simulink model "fdatool8"  (Simulink 5.1)
settings: Solver=FixedStepDiscrete  StartTime=0.0  StopTime=0.5  RelTol=1e-3
libraries: dspsigops x8, fixpt_lib_4 x8
settings Model: Creator=svenhoffmann  LastModifiedBy=svenhoffmann  ExtModeAutoUpdateStatusClock=off  BooleanDataType=on  ProdHWDeviceType=Microprocessor

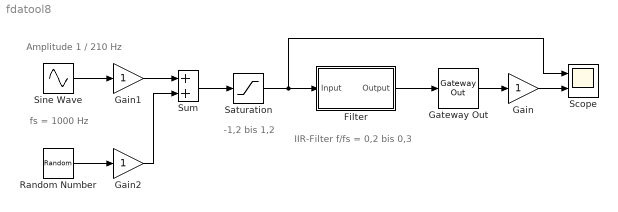
== system fdatool8 ==
  note: IIR-Filter
      | f/fs = 0,2 bis 0,3
  note: Amplitude 1 / 210 Hz
  note: fs = 1000 Hz
  note: -1,2 bis 1,2
  Filter : Subsystem  Tag=FilterWizardSubSystem
  Gain : Gain  SaturateOnIntegerOverflow=on
  Gain1 : Gain  SaturateOnIntegerOverflow=on
  Gain2 : Gain  SaturateOnIntegerOverflow=on
  Gateway Out : fixpt_lib_4/Data Type/Gateway Out  OutRealWorld=Real World Value  OutBuiltInType=double  DoSatur=off
  Random Number : RandomNumber  SampleTime=1/1000
  Saturation : Saturate  UpperLimit=1.2  LowerLimit=-1.2
  Scope : Scope  NumInputPorts=2
      settings: YMin=-5~-5  YMax=5~5
  Sine Wave : Sin  Frequency=2*pi*230  SampleTime=1/1000
  Sum : Sum  SaturateOnIntegerOverflow=on
  wires:
  Sine Wave/1 -> Gain1/1
  Gain/1 -> Scope/2
  Gateway Out/1 -> Gain/1
  Gain1/1 -> Sum/1
  Sum/1 -> Saturation/1
  Random Number/1 -> Gain2/1
  Gain2/1 -> Sum/2
  Saturation/1 -> Scope/1, Filter/1(Input)
  Filter/1(Output) -> Gateway Out/1

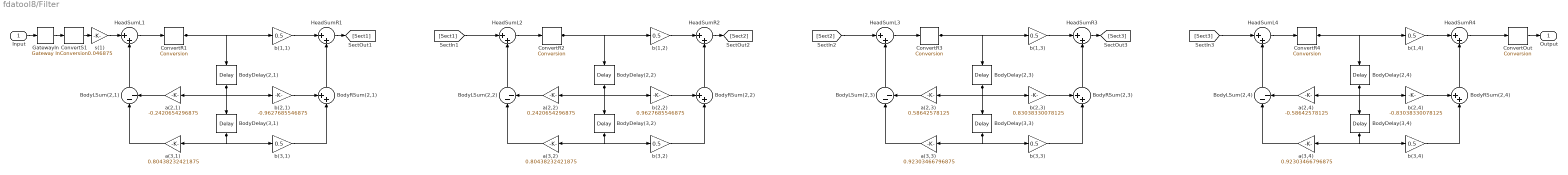
== system fdatool8/Filter ==
  Input : Inport
  BodyDelay(2,1) : dspsigops/Delay  Orientation=down  dly_unit=Samples  delay=1  ic_detail=off  dif_ic_for_ch=off  dif_ic_for_dly=off  ic=0  reset_popup=None
  BodyDelay(2,2) : dspsigops/Delay  Orientation=down  dly_unit=Samples  delay=1  ic_detail=off  dif_ic_for_ch=off  dif_ic_for_dly=off  ic=0  reset_popup=None
  BodyDelay(2,3) : dspsigops/Delay  Orientation=down  dly_unit=Samples  delay=1  ic_detail=off  dif_ic_for_ch=off  dif_ic_for_dly=off  ic=0  reset_popup=None
  BodyDelay(2,4) : dspsigops/Delay  Orientation=down  dly_unit=Samples  delay=1  ic_detail=off  dif_ic_for_ch=off  dif_ic_for_dly=off  ic=0  reset_popup=None
  BodyDelay(3,1) : dspsigops/Delay  Orientation=down  dly_unit=Samples  delay=1  ic_detail=off  dif_ic_for_ch=off  dif_ic_for_dly=off  ic=0  reset_popup=None
  BodyDelay(3,2) : dspsigops/Delay  Orientation=down  dly_unit=Samples  delay=1  ic_detail=off  dif_ic_for_ch=off  dif_ic_for_dly=off  ic=0  reset_popup=None
  BodyDelay(3,3) : dspsigops/Delay  Orientation=down  dly_unit=Samples  delay=1  ic_detail=off  dif_ic_for_ch=off  dif_ic_for_dly=off  ic=0  reset_popup=None
  BodyDelay(3,4) : dspsigops/Delay  Orientation=down  dly_unit=Samples  delay=1  ic_detail=off  dif_ic_for_ch=off  dif_ic_for_dly=off  ic=0  reset_popup=None
  BodyLSum(2,1) : Sum  Orientation=up  Inputs=|--  ShowAdditionalParam=on  OutDataTypeMode=Specify via dialog  OutDataType=sfix(32)  OutScaling=2^-28  SaturateOnIntegerOverflow=on  LockScale=on
  BodyLSum(2,2) : Sum  Orientation=up  Inputs=|--  ShowAdditionalParam=on  OutDataTypeMode=Specify via dialog  OutDataType=sfix(32)  OutScaling=2^-28  SaturateOnIntegerOverflow=on  LockScale=on
  BodyLSum(2,3) : Sum  Orientation=up  Inputs=|--  ShowAdditionalParam=on  OutDataTypeMode=Specify via dialog  OutDataType=sfix(32)  OutScaling=2^-28  SaturateOnIntegerOverflow=on  LockScale=on
  BodyLSum(2,4) : Sum  Orientation=up  Inputs=|--  ShowAdditionalParam=on  OutDataTypeMode=Specify via dialog  OutDataType=sfix(32)  OutScaling=2^-28  SaturateOnIntegerOverflow=on  LockScale=on
  BodyRSum(2,1) : Sum  Orientation=up  Inputs=++|  ShowAdditionalParam=on  OutDataTypeMode=Specify via dialog  OutDataType=sfix(32)  OutScaling=2^-28  SaturateOnIntegerOverflow=on  LockScale=on
  BodyRSum(2,2) : Sum  Orientation=up  Inputs=++|  ShowAdditionalParam=on  OutDataTypeMode=Specify via dialog  OutDataType=sfix(32)  OutScaling=2^-28  SaturateOnIntegerOverflow=on  LockScale=on
  BodyRSum(2,3) : Sum  Orientation=up  Inputs=++|  ShowAdditionalParam=on  OutDataTypeMode=Specify via dialog  OutDataType=sfix(32)  OutScaling=2^-28  SaturateOnIntegerOverflow=on  LockScale=on
  BodyRSum(2,4) : Sum  Orientation=up  Inputs=++|  ShowAdditionalParam=on  OutDataTypeMode=Specify via dialog  OutDataType=sfix(32)  OutScaling=2^-28  SaturateOnIntegerOverflow=on  LockScale=on
  ConvertOut : fixpt_lib_4/Data Type/Conversion  ConvertRealWorld=Real World Value  OutputDataTypeScalingMode=Specify via dialog  OutDataType=sfix(16)  OutScaling=2^-14  DoSatur=on
      settings: LockScale=on
  ConvertR{1..4} (4 alike) : fixpt_lib_4/Data Type/Conversion  ConvertRealWorld=Real World Value  OutputDataTypeScalingMode=Specify via dialog  OutDataType=sfix(16)  OutScaling=2^-14  DoSatur=on
      settings: LockScale=on
  ConvertS1 : fixpt_lib_4/Data Type/Conversion  ConvertRealWorld=Real World Value  OutputDataTypeScalingMode=Specify via dialog  OutDataType=sfix(16)  OutScaling=2^-14  DoSatur=on
      settings: LockScale=on
  GatewayIn : fixpt_lib_4/Data Type/Gateway In  InRealWorld=Real World Value  OutputDataTypeScalingMode=Specify via dialog  OutDataType=sfix(16)  OutScaling=2^-14  DoSatur=on
      settings: LockScale=on
  HeadSumL{1..4} (4 alike) : Sum  Inputs=|++  ShowAdditionalParam=on  OutDataTypeMode=Specify via dialog  OutDataType=sfix(32)  OutScaling=2^-28  SaturateOnIntegerOverflow=on  LockScale=on
  HeadSumR{1..4} (4 alike) : Sum  Inputs=|++  ShowAdditionalParam=on  OutDataTypeMode=Specify via dialog  OutDataType=sfix(32)  OutScaling=2^-28  SaturateOnIntegerOverflow=on  LockScale=on
  a(2,1) : Gain  Orientation=left  Gain=-0.2420654296875  ShowAdditionalParam=on  ParameterDataTypeMode=Specify via dialog  ParameterScalingMode=Use specified scaling  ParameterScaling=2^-14  OutDataTypeMode=Specify via dialog  OutDataType=sfix(32)  OutScaling=2^-28  SaturateOnIntegerOverflow=on  LockScale=on
  a(2,2) : Gain  Orientation=left  Gain=0.2420654296875  ShowAdditionalParam=on  ParameterDataTypeMode=Specify via dialog  ParameterScalingMode=Use specified scaling  ParameterScaling=2^-14  OutDataTypeMode=Specify via dialog  OutDataType=sfix(32)  OutScaling=2^-28  SaturateOnIntegerOverflow=on  LockScale=on
  a(2,3) : Gain  Orientation=left  Gain=0.58642578125  ShowAdditionalParam=on  ParameterDataTypeMode=Specify via dialog  ParameterScalingMode=Use specified scaling  ParameterScaling=2^-14  OutDataTypeMode=Specify via dialog  OutDataType=sfix(32)  OutScaling=2^-28  SaturateOnIntegerOverflow=on  LockScale=on
  a(2,4) : Gain  Orientation=left  Gain=-0.58642578125  ShowAdditionalParam=on  ParameterDataTypeMode=Specify via dialog  ParameterScalingMode=Use specified scaling  ParameterScaling=2^-14  OutDataTypeMode=Specify via dialog  OutDataType=sfix(32)  OutScaling=2^-28  SaturateOnIntegerOverflow=on  LockScale=on
  a(3,1) : Gain  Orientation=left  Gain=0.80438232421875  ShowAdditionalParam=on  ParameterDataTypeMode=Specify via dialog  ParameterScalingMode=Use specified scaling  ParameterScaling=2^-14  OutDataTypeMode=Specify via dialog  OutDataType=sfix(32)  OutScaling=2^-28  SaturateOnIntegerOverflow=on  LockScale=on
  a(3,2) : Gain  Orientation=left  Gain=0.80438232421875  ShowAdditionalParam=on  ParameterDataTypeMode=Specify via dialog  ParameterScalingMode=Use specified scaling  ParameterScaling=2^-14  OutDataTypeMode=Specify via dialog  OutDataType=sfix(32)  OutScaling=2^-28  SaturateOnIntegerOverflow=on  LockScale=on
  a(3,3) : Gain  Orientation=left  Gain=0.92303466796875  ShowAdditionalParam=on  ParameterDataTypeMode=Specify via dialog  ParameterScalingMode=Use specified scaling  ParameterScaling=2^-14  OutDataTypeMode=Specify via dialog  OutDataType=sfix(32)  OutScaling=2^-28  SaturateOnIntegerOverflow=on  LockScale=on
  a(3,4) : Gain  Orientation=left  Gain=0.92303466796875  ShowAdditionalParam=on  ParameterDataTypeMode=Specify via dialog  ParameterScalingMode=Use specified scaling  ParameterScaling=2^-14  OutDataTypeMode=Specify via dialog  OutDataType=sfix(32)  OutScaling=2^-28  SaturateOnIntegerOverflow=on  LockScale=on
  b(1,1) : Gain  Gain=0.5  ShowAdditionalParam=on  ParameterDataTypeMode=Specify via dialog  ParameterScalingMode=Use specified scaling  ParameterScaling=2^-14  OutDataTypeMode=Specify via dialog  OutDataType=sfix(32)  OutScaling=2^-28  SaturateOnIntegerOverflow=on  LockScale=on
  b(1,2) : Gain  Gain=0.5  ShowAdditionalParam=on  ParameterDataTypeMode=Specify via dialog  ParameterScalingMode=Use specified scaling  ParameterScaling=2^-14  OutDataTypeMode=Specify via dialog  OutDataType=sfix(32)  OutScaling=2^-28  SaturateOnIntegerOverflow=on  LockScale=on
  b(1,3) : Gain  Gain=0.5  ShowAdditionalParam=on  ParameterDataTypeMode=Specify via dialog  ParameterScalingMode=Use specified scaling  ParameterScaling=2^-14  OutDataTypeMode=Specify via dialog  OutDataType=sfix(32)  OutScaling=2^-28  SaturateOnIntegerOverflow=on  LockScale=on
  b(1,4) : Gain  Gain=0.5  ShowAdditionalParam=on  ParameterDataTypeMode=Specify via dialog  ParameterScalingMode=Use specified scaling  ParameterScaling=2^-14  OutDataTypeMode=Specify via dialog  OutDataType=sfix(32)  OutScaling=2^-28  SaturateOnIntegerOverflow=on  LockScale=on
  b(2,1) : Gain  Gain=-0.9627685546875  ShowAdditionalParam=on  ParameterDataTypeMode=Specify via dialog  ParameterScalingMode=Use specified scaling  ParameterScaling=2^-14  OutDataTypeMode=Specify via dialog  OutDataType=sfix(32)  OutScaling=2^-28  SaturateOnIntegerOverflow=on  LockScale=on
  b(2,2) : Gain  Gain=0.9627685546875  ShowAdditionalParam=on  ParameterDataTypeMode=Specify via dialog  ParameterScalingMode=Use specified scaling  ParameterScaling=2^-14  OutDataTypeMode=Specify via dialog  OutDataType=sfix(32)  OutScaling=2^-28  SaturateOnIntegerOverflow=on  LockScale=on
  b(2,3) : Gain  Gain=0.83038330078125  ShowAdditionalParam=on  ParameterDataTypeMode=Specify via dialog  ParameterScalingMode=Use specified scaling  ParameterScaling=2^-14  OutDataTypeMode=Specify via dialog  OutDataType=sfix(32)  OutScaling=2^-28  SaturateOnIntegerOverflow=on  LockScale=on
  b(2,4) : Gain  Gain=-0.83038330078125  ShowAdditionalParam=on  ParameterDataTypeMode=Specify via dialog  ParameterScalingMode=Use specified scaling  ParameterScaling=2^-14  OutDataTypeMode=Specify via dialog  OutDataType=sfix(32)  OutScaling=2^-28  SaturateOnIntegerOverflow=on  LockScale=on
  b(3,1) : Gain  Gain=0.5  ShowAdditionalParam=on  ParameterDataTypeMode=Specify via dialog  ParameterScalingMode=Use specified scaling  ParameterScaling=2^-14  OutDataTypeMode=Specify via dialog  OutDataType=sfix(32)  OutScaling=2^-28  SaturateOnIntegerOverflow=on  LockScale=on
  b(3,2) : Gain  Gain=0.5  ShowAdditionalParam=on  ParameterDataTypeMode=Specify via dialog  ParameterScalingMode=Use specified scaling  ParameterScaling=2^-14  OutDataTypeMode=Specify via dialog  OutDataType=sfix(32)  OutScaling=2^-28  SaturateOnIntegerOverflow=on  LockScale=on
  b(3,3) : Gain  Gain=0.5  ShowAdditionalParam=on  ParameterDataTypeMode=Specify via dialog  ParameterScalingMode=Use specified scaling  ParameterScaling=2^-14  OutDataTypeMode=Specify via dialog  OutDataType=sfix(32)  OutScaling=2^-28  SaturateOnIntegerOverflow=on  LockScale=on
  b(3,4) : Gain  Gain=0.5  ShowAdditionalParam=on  ParameterDataTypeMode=Specify via dialog  ParameterScalingMode=Use specified scaling  ParameterScaling=2^-14  OutDataTypeMode=Specify via dialog  OutDataType=sfix(32)  OutScaling=2^-28  SaturateOnIntegerOverflow=on  LockScale=on
  s(1) : Gain  Gain=0.046875  ShowAdditionalParam=on  ParameterDataTypeMode=Specify via dialog  ParameterScalingMode=Use specified scaling  ParameterScaling=2^-14  OutDataTypeMode=Specify via dialog  OutDataType=sfix(32)  OutScaling=2^-28  SaturateOnIntegerOverflow=on  LockScale=on
  Output : Outport
  wires:
  s(1)/1 -> HeadSumL1/1
  b(1,1)/1 -> HeadSumR1/1
  HeadSumR1/1 -> [Sect1]
  BodyDelay(2,1)/1 -> a(2,1)/1, b(2,1)/1, BodyDelay(3,1)/1
  a(2,1)/1 -> BodyLSum(2,1)/2
  b(2,1)/1 -> BodyRSum(2,1)/1
  BodyLSum(2,1)/1 -> HeadSumL1/2
  BodyRSum(2,1)/1 -> HeadSumR1/2
  BodyDelay(3,1)/1 -> a(3,1)/1, b(3,1)/1
  a(3,1)/1 -> BodyLSum(2,1)/1
  b(3,1)/1 -> BodyRSum(2,1)/2
  [Sect1] -> HeadSumL2/1
  b(1,2)/1 -> HeadSumR2/1
  HeadSumR2/1 -> [Sect2]
  BodyDelay(2,2)/1 -> a(2,2)/1, b(2,2)/1, BodyDelay(3,2)/1
  a(2,2)/1 -> BodyLSum(2,2)/2
  b(2,2)/1 -> BodyRSum(2,2)/1
  BodyLSum(2,2)/1 -> HeadSumL2/2
  BodyRSum(2,2)/1 -> HeadSumR2/2
  BodyDelay(3,2)/1 -> a(3,2)/1, b(3,2)/1
  a(3,2)/1 -> BodyLSum(2,2)/1
  b(3,2)/1 -> BodyRSum(2,2)/2
  [Sect2] -> HeadSumL3/1
  b(1,3)/1 -> HeadSumR3/1
  HeadSumR3/1 -> [Sect3]
  BodyDelay(2,3)/1 -> a(2,3)/1, b(2,3)/1, BodyDelay(3,3)/1
  a(2,3)/1 -> BodyLSum(2,3)/2
  b(2,3)/1 -> BodyRSum(2,3)/1
  BodyLSum(2,3)/1 -> HeadSumL3/2
  BodyRSum(2,3)/1 -> HeadSumR3/2
  BodyDelay(3,3)/1 -> a(3,3)/1, b(3,3)/1
  a(3,3)/1 -> BodyLSum(2,3)/1
  b(3,3)/1 -> BodyRSum(2,3)/2
  [Sect3] -> HeadSumL4/1
  b(1,4)/1 -> HeadSumR4/1
  BodyDelay(2,4)/1 -> a(2,4)/1, b(2,4)/1, BodyDelay(3,4)/1
  a(2,4)/1 -> BodyLSum(2,4)/2
  b(2,4)/1 -> BodyRSum(2,4)/1
  BodyLSum(2,4)/1 -> HeadSumL4/2
  BodyRSum(2,4)/1 -> HeadSumR4/2
  BodyDelay(3,4)/1 -> a(3,4)/1, b(3,4)/1
  a(3,4)/1 -> BodyLSum(2,4)/1
  b(3,4)/1 -> BodyRSum(2,4)/2
  ConvertS1/1 -> s(1)/1
  HeadSumL1/1 -> ConvertR1/1
  ConvertR1/1 -> BodyDelay(2,1)/1, b(1,1)/1
  HeadSumL2/1 -> ConvertR2/1
  ConvertR2/1 -> BodyDelay(2,2)/1, b(1,2)/1
  HeadSumL3/1 -> ConvertR3/1
  ConvertR3/1 -> BodyDelay(2,3)/1, b(1,3)/1
  HeadSumL4/1 -> ConvertR4/1
  ConvertR4/1 -> BodyDelay(2,4)/1, b(1,4)/1
  HeadSumR4/1 -> ConvertOut/1
  ConvertOut/1 -> Output/1
  Input/1 -> GatewayIn/1
  GatewayIn/1 -> ConvertS1/1
